simulink library "bcm"  (R2021b)
settings: Solver=VariableStepAuto  StartTime=0.0  StopTime=10.0  RelTol=1e-3
undefined symbols (not defined in the file): ENUM_ANTITHEFT_ALARM, ENUM_ANTITHEFT_ARM, ENUM_ANTITHEFT_DISARM, ENUM_ANTITHEFT_WAIT, ENUM_GEARPOSNTOCAN_P, ENUM_PDKEYRAWLULOCK_INUNLOCK, ENUM_PDKEYRAWPS_INPS, ENUM_POWERSTA_ON, ENUM_POWERSTA_READY, ENUM_POWERSTA_STANDBY, ENUM_PWRSTASW_ON, ENUM_PWRSTASW_READY, ENUM_SYSMODE_DEVELOPING, ENUM_SYSMODE_PRODUCT, ENUM_VEHICLETYPE_D21, ENUM_VEHICLETYPE_D31F25, ENUM_VEHICLETYPE_D31HAWD, ENUM_VEHICLETYPE_D31HRWD, ENUM_VEHICLETYPE_D31L24, FALSE, KBCM_ACCSwcPrsTmr_s, KBCM_ALMBrightnessDark_enum, KBCM_AmbBlue_enum, KBCM_AmbBreathT_ms, KBCM_AmbGreen_enum, KBCM_AmbMidPple_enum, KBCM_AmbRed_enum, KBCM_AmbTempCtrlEN_flg, KBCM_AmbTempT_s, KBCM_AmbWelModeENWait_s, KBCM_Antitheft_enum_ovrdflg, KBCM_Antitheft_enum_ovrdval, KBCM_APMDoorCtrlSta_flg_ovrdflg, KBCM_APMDoorCtrlSta_flg_ovrdval, KBCM_CmdKeepT_s, KBCM_CSWLightRstDebT_s, KBCM_CSWTurnLPRstT_s, KBCM_CycleTimeSet_s, KBCM_DelayTSW_flg, KBCM_DiagDRLOFF_flg, KBCM_DiagFLTC_mA, KBCM_DiagFMHT_s, KBCM_DiagFRTC_mA, KBCM_DiagRLTC_mA, KBCM_DiagRRTC_mA, KBCM_DrAPMRetryTimes_cnt, KBCM_DrOpenWdwOT_s, KBCM_DrOpenWdwReady_s, KBCM_DutyCycleSet_cnt, KBCM_DutyOverride_flg, KBCM_DutyOverride_val, KBCM_ESSOffT_ms, KBCM_ESSOnT_ms, KBCM_FDCDKCReDetectT_K, KBCM_FDCDKCUSSFilterT_K, KBCM_HandleLampKeepT_s, KBCM_IVIRstHoldT_ms, KBCM_IVIRstTriggerT_ms, KBCM_ONDelayT_ms, KBCM_RAPSAbnFlashOFFT_ms ... (+51)
libraries: simulink x402, $bdroot x10, hcu_lib x2
(part 12 of 14)

== stateflow chart bcm/BCM/BCM/AntiTheft/Chart ==
  settings: sampleTime=StepSize
  state AlertTone [parallel]
    settings: executionOrder=11
    state OFF
      en:VBCM_LockAlarm_enum=0;
    state Lock_Success
      en:VBCM_LockAlarm_enum=1;
    (default) -> AlertTone.OFF
    Lock_Success -> AlertTone.OFF : [after(5,tick)]
    AlertTone -> Lock_Success : eLockAlert [IVI_Lock_SoundSW_Sta==1]
  state HoodRelease [parallel]
    settings: executionOrder=12
    state OFF
      en:FDC_BCM_HoodRel_Cmd=0;
    state Hood_Release
      en:FDC_BCM_HoodRel_Cmd=1;
    (default) -> HoodRelease.OFF
    (junction 2202) -> HoodRelease.OFF
    HoodRelease -> Hood_Release [order 1] : eHoodRel
        | [VehSpeed<=0 && ShiftGearPosn == ENUM_GEARPOSNTOCAN_P]
    Hood_Release -> (junction 2202) : [after(10,tick)]
    HoodRelease -> Hood_Release [order 2] : [VBCM_IVIFrTrunkUnlockReqRising_flg && ....
        | (VehSpeed<=0 && ShiftGearPosn == ENUM_GEARPOSNTOCAN_P && !DrLockSta)]
  state ATLockCtrl [parallel]
    settings: executionOrder=6
    state Lock
      en:ATLockCtrl=1;
    state StandBy
      en:ATLockCtrl=0;
    note: 350 ms
    state Unlock
      en:ATLockCtrl=2;
    (default) -> ATLockCtrl.StandBy
    ATLockCtrl.StandBy -> ATLockCtrl.Lock [order 1] : eActLock
    ATLockCtrl.Lock -> ATLockCtrl.StandBy : [after(35,tick)]
    ATLockCtrl.Unlock -> ATLockCtrl.Lock [order 2] : eActLock
    ATLockCtrl.StandBy -> ATLockCtrl.Unlock [order 2] : eActUnlock
    ATLockCtrl.Unlock -> ATLockCtrl.StandBy [order 1] : [after(35,tick)]
  state Main [parallel]
    settings: executionOrder=1
    state sDisarm
      en:AntitheftSta=0;
      fFirst=1;
    state sSecurity
      state sSecurity
        en:
        AntitheftSta=1;
        fFirst=0;
      note: 28 sec
      note: 10 times
      state sAlarm
        en:
        AntitheftSta=3;
        ATAlarm=1;
        Horn.eHornAlarm;
        CountAlarm=CountAlarm+1;
        ex:ATAlarm=0;
      (junction 1705) -> (junction 1971) [order 2] : {Horn.eHornLock;}
      (junction 1705) -> Main.sSecurity.sSecurity [order 1] : [fHornOFF==1||fFirst==1]
          | /{fHornOFF=0;AlertTone.eLockAlert;}
      (junction 1971) -> Main.sSecurity.sSecurity
      Main.sSecurity.sSecurity -> sAlarm : eDoorOpen[CountAlarm<10]
      sAlarm -> Main.sSecurity.sSecurity : [after(2800,tick)]
    note: 1 sec
    state sLockCheck
    (default) -> (junction 2132) : {CountAlarm = VINP_FlashCountAlarm_enum;}
    (junction 2132) -> (junction 2133) [order 1]
    (junction 2133) -> (junction 2135) [order 1]
    (junction 2132) -> sDisarm [order 2]
    (junction 2133) -> Main.sSecurity.sSecurity [order 2] : [VBCM_FlashAntitheft_enum == ENUM_ANTITHEFT_ARM]
    (junction 2135) -> sAlarm : [VBCM_FlashAntitheft_enum == ENUM_ANTITHEFT_ALARM]
    (junction 1713) -> sDisarm : {ATLockCtrl.eActUnlock;Horn.eLockFail;}
    (junction 1703) -> (junction 1713) [order 1] : [!DrLockSta||AllDoorSW||TailgateSW||HoodSW]
    (junction 1703) -> (junction 1705) [order 2] : {CountAlarm=0;}
    (junction 1686) -> (junction 1713) [order 1] : [AllDoorSW||TailgateSW||HoodSW]
    sLockCheck -> (junction 1703) : [after(100,tick)]
    sDisarm -> sDisarm [order 2] : eUnlock{ATCtrl.eLampUnlock;ATLockCtrl.eActUnlock;}
    (junction 1686) -> sLockCheck [order 2] : {ATLockCtrl.eActLock;}
    (junction 1712) -> (junction 1686) : {ATCtrl.eLampLock;}
    sDisarm -> (junction 1712) [order 1] : eLock
    Main.sSecurity -> (junction 1712) [order 2] : eLock
    Main.sSecurity -> sDisarm [order 1] : eUnlock{ATCtrl.eLampUnlock;ATLockCtrl.eActUnlock;}
    Main.sSecurity -> sDisarm [order 3] : eForceDisarm
  state DKCCmd [parallel]
    settings: executionOrder=2
    state WaitForZone
    state Lock
      en:Main.eLock;
    state Unlock
      en:Main.eUnlock;
    state sStandBy
    state Tailgate
      en:DoorSWDetection.TailgateSW.eTailgate;
      PowerTailgate.eTailgateRemote;
    state FindCar
      en:Horn.eHornLock;ATCtrl.eLampUnlock;
    state TailgateLockFail
      en:Horn.eLockFail;Main.eUnlock;
    state TailgateHandle
      en:DoorSWDetection.TailgateSW.eTailgate;
      PowerTailgate.eTailgateHandle;
    state ForceDisarm
      en:Main.eForceDisarm;
    state FindCarMute
      en:ATCtrl.eLampUnlock;
    state HoodRel
      en:HoodRelease.eHoodRel;
      DoorSWDetection.HoodSW.eHoodRemote;
    DKCCmd -> (junction 2148) : [hasChanged(P_CommandtoBCM)]{PcmdBuf=P_CommandtoBCM;}
    (junction 2148) -> DKCCmd.WaitForZone [order 2]
    (junction 2148) -> (junction 2154) [order 1]
    DKCCmd.WaitForZone -> (junction 2154) [order 2]
    (junction 2154) -> (junction 2045) : [VINP_CANMsgValidGWZoneDR1_flg&&VINP_CANMsgValidGWZoneFR1_flg && Loadbar]
    DKCCmd.WaitForZone -> (junction 2151) [order 1] : [after(150,tick)]
    (junction 2151) -> (junction 2045)
    (junction 2045) -> (junction 2170) [order 1] : [VehSpeed<=0]
    (junction 2170) -> DKCCmd.Lock [order 1] : [PcmdBuf==1]
    (junction 2045) -> (junction 2046) [order 2]
    (junction 2170) -> (junction 2172) [order 2]
    (junction 2172) -> DKCCmd.Lock [order 1] : [PcmdBuf==10 &&....
        | FDC_BCM_WalkOutLkEnFun_Sta==1]
    (junction 2172) -> (junction 2178) [order 2]
    (junction 2178) -> (junction 2180) [order 1] : [PcmdBuf==9]
    (junction 2180) -> DKCCmd.Lock [order 1] : [AntitheftSta==0]
    (junction 2178) -> (junction 2186) [order 2]
    (junction 2180) -> (junction 2183) [order 2]
    (junction 2183) -> DKCCmd.Unlock
    (junction 2186) -> DKCCmd.Unlock [order 1] : [PcmdBuf==11 &&....
        | FDC_BCM_WalkInUnLkEnFun_Sta==1]
    (junction 2186) -> (junction 2189) [order 2]
    (junction 2189) -> DKCCmd.Unlock : [PcmdBuf==2]
    (junction 2046) -> DKCCmd.Unlock [order 1] : [VehSpeed<=0&&PcmdBuf==2]
    (junction 2046) -> (junction 2047) [order 2]
    (default) -> DKCCmd.sStandBy : {PcmdBuf=0;}
    (junction 2047) -> DKCCmd.Tailgate [order 1] : [PcmdBuf==3]
    (junction 2047) -> (junction 2048) [order 2]
    (junction 2048) -> DKCCmd.FindCar [order 1] : [PcmdBuf==4]
    (junction 2048) -> (junction 2049) [order 2]
    (junction 2049) -> TailgateLockFail [order 1] : [PcmdBuf==5]
    (junction 2049) -> (junction 2050) [order 2]
    (junction 2050) -> DKCCmd.TailgateHandle [order 1] : [PcmdBuf==6]
    (junction 2050) -> (junction 2108) [order 2]
    (junction 2108) -> ForceDisarm [order 1] : [PcmdBuf==7]
    (junction 2108) -> (junction 2124) [order 2]
    (junction 2124) -> DKCCmd.FindCarMute [order 1] : [PcmdBuf==8]
    (junction 2124) -> (junction 2193) [order 2]
    (junction 2193) -> DKCCmd.sStandBy [order 2]
    (junction 2193) -> DKCCmd.HoodRel [order 1] : [PcmdBuf==12]
  state Horn [parallel]
    settings: executionOrder=3
    state sStandBy
      en:HornCtrl=0;
    note: 250 ms
    state sAlarm2
      en:HornCtrl=0;
    state sAlarm1
      en:HornCtrl=1;
    state sLock
      en:HornCtrl=1;
    state sKeyIN1
      en:HornCtrl=1;
    state sKeyIN2
      en:HornCtrl=0;
    state sLockFail1
      en:HornCtrl=1;
    state sLockFail2
      en:HornCtrl=0;
    state sLockFail3
      en:HornCtrl=1;
    state sRAPSAlarm2
      en:HornCtrl=0;
    state sRAPSAlarm1
      en:HornCtrl=1;
    (default) -> Horn.sStandBy
    (junction 2243) -> Horn.sStandBy
    sAlarm1 -> sAlarm2 : [after(25,tick)]
    sAlarm2 -> (junction 2243) [order 1] : [ATAlarm==0]
    Horn -> sAlarm1 [order 1] : eHornAlarm
    (junction 2244) -> (junction 2243)
    sAlarm2 -> sAlarm1 [order 2] : [after(25,tick)]
    sLock -> (junction 2244) : [after(3,tick)]
    (junction 2245) -> (junction 2244)
    Horn -> sLock [order 2] : eHornLock
    sKeyIN2 -> sLock : [after(5,tick)]
    Horn -> sKeyIN1 [order 3] : eKeyIN
    sKeyIN1 -> sKeyIN2 : [after(3,tick)]
    Horn -> sLockFail1 [order 4] : eLockFail
    sLockFail1 -> sLockFail2 : [after(10,tick)]
    sLockFail2 -> sLockFail3 : [after(30,tick)]
    sLockFail3 -> (junction 2245) : [after(10,tick)]
    (junction 2246) -> (junction 2245)
    sRAPSAlarm1 -> sRAPSAlarm2 : [after(25,tick)]
    sRAPSAlarm2 -> (junction 2246) [order 2] : [RAPSHornReq==0]
    Horn -> sRAPSAlarm1 [order 5] : eRAPSHorn
    sRAPSAlarm2 -> sRAPSAlarm1 [order 1] : [after(25,tick)]
  state DoorSWDetection [parallel]
    settings: executionOrder=4
    state DrDoor [parallel]
      settings: executionOrder=1
      state DrDoorSW_Open
      state DrDoorSW_Close
      (default) -> DrDoorSW_Open
      DrDoorSW_Open -> DrDoorSW_Close : [!DrDoorSW]
      DrDoorSW_Close -> DrDoorSW_Open : [DrDoorSW]/{Main.eDoorOpen;}
    state PsDoor [parallel]
      settings: executionOrder=2
      state PsDoorSW_Open
      state PsDoorSW_Close
      (default) -> PsDoorSW_Open
      PsDoorSW_Open -> PsDoorSW_Close : [!PsDoorSW]
      PsDoorSW_Close -> PsDoorSW_Open : [PsDoorSW]/{Main.eDoorOpen;}
    state RLDoor [parallel]
      settings: executionOrder=3
      state RLDoorSW_Open
      state RLDoorSW_Close
      (default) -> RLDoorSW_Open
      RLDoorSW_Open -> RLDoorSW_Close : [!RLDoorSW]
      RLDoorSW_Close -> RLDoorSW_Open : [RLDoorSW]/{Main.eDoorOpen;}
    state RRDoor [parallel]
      settings: executionOrder=4
      state RRDoorSW_Open
      state RRDoorSW_Close
      (default) -> RRDoorSW_Open
      RRDoorSW_Open -> RRDoorSW_Close : [!RRDoorSW]
      RRDoorSW_Close -> RRDoorSW_Open : [RRDoorSW]/{Main.eDoorOpen;}
    state HoodSW [parallel]
      settings: executionOrder=6
      state HoodSW_Open
      state HoodSW_Close
      state sRemote
      state Wait
      state Ignore
      (default) -> HoodSW_Open
      HoodSW_Open -> HoodSW_Close : [!HoodSW]
      HoodSW_Close -> HoodSW_Open [order 1] : [HoodSW]/{Main.eDoorOpen;}
      HoodSW_Close -> DoorSWDetection.HoodSW.sRemote [order 2] : eHoodRemote
      (junction 2220) -> HoodSW_Close [order 2] : [after(2000,tick)]
      Wait -> HoodSW_Close [order 2] : after(100,tick)
      DoorSWDetection.HoodSW.sRemote -> (junction 2220)
      (junction 2220) -> DoorSWDetection.HoodSW.Ignore [order 1] : [HoodSW]
      Wait -> DoorSWDetection.HoodSW.Ignore [order 1] : [HoodSW]
      DoorSWDetection.HoodSW.Ignore -> Wait : [!HoodSW]
    note: 20 sec
    state TailgateSW [parallel]
      settings: executionOrder=5
      state TailgateSW_Open
      state TailgateSW_Close
      state sRemote
      state Ignore
      (default) -> TailgateSW_Open
      TailgateSW_Open -> TailgateSW_Close : [!TailgateSW]
      TailgateSW_Close -> TailgateSW_Open [order 1] : [TailgateSW]/{Main.eDoorOpen;}
      TailgateSW_Close -> DoorSWDetection.TailgateSW.sRemote [order 2] : eTailgate
      (junction 1886) -> TailgateSW_Close [order 2] : [after(1500,tick)]
      DoorSWDetection.TailgateSW.Ignore -> TailgateSW_Close : [!TailgateSW]
      DoorSWDetection.TailgateSW.sRemote -> (junction 1886)
      (junction 1886) -> DoorSWDetection.TailgateSW.Ignore [order 1] : [TailgateSW]
    note: 15 sec
  state VIGCommand [parallel]
    settings: executionOrder=7
    state WaitForZone
    state StandBy
    state Lock
      en:Main.eLock;
    state Unlock
      en:Main.eUnlock;
    state FindCar
      en:Horn.eHornLock;ATCtrl.eLampUnlock;
    state FindCarMute
      en:ATCtrl.eLampUnlock;
    state Tailgate
      en:DoorSWDetection.TailgateSW.eTailgate;
      PowerTailgate.eTailgateRemote;
    state TailgateReject
      en:PowerTailgate.eTailgateReject;
    state HoodRel
      en:HoodRelease.eHoodRel;
      DoorSWDetection.HoodSW.eHoodRemote;
    (default) -> VIGCommand.WaitForZone
    VIGCommand.WaitForZone -> VIGCommand.StandBy : [VINP_CANMsgValidGWZoneDR1_flg&&VINP_CANMsgValidGWZoneFR1_flg]
    VIGCommand.StandBy -> VIGCommand.Lock [order 1] : [VehSpeed<=0&&(VIG_Cmd==1||VIG_Cmd==5)]
    VIGCommand.Lock -> VIGCommand.StandBy : [VIG_Cmd==0]
    (junction 1941) -> VIGCommand.Lock [order 1] : [AntitheftSta==0||AntitheftSta==2]/{fHornOFF=1;}
    VIGCommand.StandBy -> (junction 1941) [order 6] : [VehSpeed<=0&&VIG_Cmd==7]
    (junction 1941) -> VIGCommand.Unlock [order 2] : [fVIGHandle==0]
    VIGCommand.StandBy -> VIGCommand.Unlock [order 2] : [VehSpeed<=0&&(VIG_Cmd==2||VIG_Cmd==6)]
    VIGCommand.Unlock -> VIGCommand.StandBy : [VIG_Cmd==0]
    VIGCommand.StandBy -> VIGCommand.FindCar [order 3] : [VIG_Cmd==3]
    VIGCommand.FindCar -> VIGCommand.StandBy : [VIG_Cmd==0]
    VIGCommand.StandBy -> VIGCommand.FindCarMute [order 5] : [VIG_Cmd==8]
    VIGCommand.FindCarMute -> VIGCommand.StandBy : [VIG_Cmd==0]
    VIGCommand.Tailgate -> VIGCommand.StandBy : [VIG_Cmd==0]
    (junction 2118) -> VIGCommand.Tailgate
    (junction 2116) -> (junction 2118) [order 2]
    VIGCommand.StandBy -> (junction 2116) [order 4] : [VIG_Cmd==4]
    (junction 2116) -> TailgateReject [order 1] : [PwrSta==5]
    TailgateReject -> VIGCommand.StandBy : [VIG_Cmd==0]
    VIGCommand.StandBy -> VIGCommand.HoodRel [order 7] : [VIG_Cmd==11]
    VIGCommand.HoodRel -> VIGCommand.StandBy : [VIG_Cmd==0]
  state PowerTailgate [parallel]
    settings: executionOrder=9
    state StandBy
      en:TailgateRemote=0;
    state TailgateRemote
      en:TailgateRemote=1;
    note: 200 ms
    state TailgateHandle
      en:TailgateRemote=2;
    note: 200 ms
    state TailgateHandle1
      en:TailgateRemote=3;
    (default) -> PowerTailgate.StandBy
    PowerTailgate.StandBy -> TailgateRemote [order 1] : eTailgateRemote
    TailgateRemote -> PowerTailgate.StandBy : [after(20,tick)]
    PowerTailgate.StandBy -> PowerTailgate.TailgateHandle [order 2] : eTailgateHandle
    PowerTailgate.TailgateHandle -> PowerTailgate.StandBy : [after(20,tick)]
    PowerTailgate.StandBy -> TailgateHandle1 [order 3] : eTailgateReject
    TailgateHandle1 -> PowerTailgate.StandBy : [after(20,tick)]
  state AGSTailgateOpen [parallel]
    settings: executionOrder=8
    state sStandBy
    state Tailgate
      en:DoorSWDetection.TailgateSW.eTailgate;
      PowerTailgate.eTailgateRemote;
    (default) -> AGSTailgateOpen.sStandBy
    AGSTailgateOpen.sStandBy -> AGSTailgateOpen.Tailgate : [APSOpenPTG==1&&TailgateSW==0]
    AGSTailgateOpen.Tailgate -> AGSTailgateOpen.sStandBy : [APSOpenPTG==0]
  state AntitheftSeat [parallel]
    settings: executionOrder=10
    state StandBy
      en:AntitheftSeatFlod=0;
    state Lock_Check
      en:AntitheftSeatFlod=0;
    state Flod
      en:AntitheftSeatFlod=1;
    note: 200 ms
    (default) -> AntitheftSeat.StandBy
    AntitheftSeat.StandBy -> Lock_Check : [fHornOFF==1]
    Lock_Check -> Flod : [fHornOFF==0]
    Flod -> Lock_Check [order 2] : [fHornOFF==1]
    Flod -> AntitheftSeat.StandBy [order 1] : [after(20,tick)]
  state RAPS_Lock_Request [parallel]
    settings: executionOrder=13
    state NOReq
    state LOCK
      en:Main.eLock;
    (default) -> RAPS_Lock_Request.NOReq
    RAPS_Lock_Request.NOReq -> LOCK : [hasChanged(RAPSBCMLockReqCmd) &&....
        | RAPSBCMLockReqCmd &&....
        | PwrSta>3]
    LOCK -> RAPS_Lock_Request.NOReq : [!RAPSBCMLockReqCmd]
  state RAPS_Horn [parallel]
    settings: executionOrder=14
    state NoRequest
      en:
      RAPSHornReq=0;
    state RAPS_HornReq
      en:
      Horn.eRAPSHorn;
      RAPSHornReq=1;
    (default) -> NoRequest
    NoRequest -> RAPS_HornReq : [DrSeatSta!=1 && hasChanged(RAPSErrWarn) && RAPSErrWarn==2]
    RAPS_HornReq -> NoRequest : [DrSeatSta==1 || RAPSErrWarn!=2 || after(2800,tick)]
  state RAPS_UnLock_Request [parallel]
    settings: executionOrder=15
    state NOReq
    state UNLOCK
      en:Main.eUnlock;
    (default) -> RAPS_UnLock_Request.NOReq
    RAPS_UnLock_Request.NOReq -> UNLOCK : [RAPS_Unlock_Req]
    UNLOCK -> RAPS_UnLock_Request.NOReq : [!RAPS_Unlock_Req]
  state ATCtrl [parallel]
    settings: executionOrder=5
    state StandBy
      en:ATCtrl=0;
    state Lock
      en:ATCtrl=1;
    note: 350 ms
    state Unlock
      en:ATCtrl=2;
    (default) -> ATCtrl.StandBy
    ATCtrl.StandBy -> ATCtrl.Lock [order 1] : eLampLock
    ATCtrl.Lock -> ATCtrl.StandBy [order 1] : [after(35,tick)]
    ATCtrl.Unlock -> ATCtrl.Lock [order 2] : eLampLock
    ATCtrl.Lock -> ATCtrl.Unlock [order 2] : eLampUnlock
    ATCtrl.StandBy -> ATCtrl.Unlock [order 2] : eLampUnlock
    ATCtrl.Unlock -> ATCtrl.StandBy [order 1] : [after(35,tick)]
  data: P_CommandtoBCM input uint8 [0..11]; PwrSta input uint8 [0..5]; ATCtrl output uint8; ATLockCtrl output uint8; AllDoorSW input boolean [0..1]; HoodSW input boolean; TailgateSW input boolean; DrDoorSW input boolean; PsDoorSW input boolean; RLDoorSW input boolean; RRDoorSW input boolean; DrLockSta input boolean; ATAlarm output boolean; AntitheftSta output uint8; TailgateRemote output uint8; HornCtrl output boolean; VIG_Cmd input uint8 [0..7]; VehSpeed input single [0..1]; fVIGHandle input boolean; VBCM_FlashAntitheft_enum input uint8; fFirst local boolean; fHornOFF local boolean; AntitheftSeatFlod output boolean; APSOpenPTG input boolean; ENUM_ANTITHEFT_ALARM parameter uint8; ENUM_ANTITHEFT_ARM parameter uint8; VINP_FlashCountAlarm_enum input uint8; VINP_CANMsgValidGWZoneDR1_flg input boolean; VINP_CANMsgValidGWZoneFR1_flg input boolean; PcmdBuf local uint8; CountAlarm output uint8; IVI_Lock_SoundSW_Sta input boolean; FDC_BCM_WalkOutLkEnFun_Sta input; FDC_BCM_WalkInUnLkEnFun_Sta input; VBCM_LockAlarm_enum output uint8; Loadbar input; ShiftGearPosn input; FDC_BCM_HoodRel_Cmd output boolean; VBCM_IVIFrTrunkUnlockReqRising_flg input; ENUM_GEARPOSNTOCAN_P parameter; DrSeatSta input; RAPSBCMLockReqCmd input; RAPSErrWarn input; RAPSHornReq local boolean; RAPS_Unlock_Req input
  data PwrSta settings: description=Min=0, Max=2047, Engineering Unit = km/h, Offset=0 km/h, Resolution= 0.125 km/h per bit, >2047 = Invalid (bit 12 = 1)
  events: eLockAlert local FUNCTION_CALL_EVENT; eHoodRel local FUNCTION_CALL_EVENT; eActLock local FUNCTION_CALL_EVENT; eActUnlock local FUNCTION_CALL_EVENT; eLock local FUNCTION_CALL_EVENT; eUnlock local FUNCTION_CALL_EVENT; eDoorOpen local FUNCTION_CALL_EVENT; eForceDisarm local FUNCTION_CALL_EVENT; eHornAlarm local FUNCTION_CALL_EVENT; eHornLock local FUNCTION_CALL_EVENT; eKeyIN local FUNCTION_CALL_EVENT; eLockFail local FUNCTION_CALL_EVENT; eRAPSHorn local FUNCTION_CALL_EVENT; eHoodRemote local FUNCTION_CALL_EVENT; eTailgate local FUNCTION_CALL_EVENT; eTailgateRemote local FUNCTION_CALL_EVENT; eTailgateHandle local FUNCTION_CALL_EVENT; eTailgateReject local FUNCTION_CALL_EVENT; eLampLock local FUNCTION_CALL_EVENT; eLampUnlock local FUNCTION_CALL_EVENT

== stateflow chart bcm/BCM/BCM/CenterDoorLock/Chart ==
  settings: updateMethod=DISCRETE
  state CrashDetect [parallel]
    settings: executionOrder=7
    state OFF [commented out]
    state KeyON [commented out]
      state Initial [commented out]
        en:
        CrashDetd=0;
      state sCrash [commented out]
        en:CrashDetd=1;Unlockreq=1;
      note: 750 ms
      state Detect [commented out]
      Initial -> Detect [commented out] : [after(75,tick)]
      Detect -> sCrash [commented out] : [CrashOutputSts>0||....
          | (CrashInputFreq>4.1&&....
          | CrashInputFreq<4.2&&....
          | CrashInputDuty>16&&....
          | CrashInputDuty<17)]
    (default) -> CrashDetect.OFF [commented out]
    CrashDetect.OFF -> Initial [commented out] : [PwrSta>3]
    KeyON -> CrashDetect.OFF [commented out] : [PwrSta<=3]
    (default) -> (junction 1980)
    (junction 1980) -> (junction 1981) : [hasChanged(CrashDetd) && CrashDetd == TRUE]
    CrashDetect -> (junction 1980)
    (junction 1981) -> (junction 1979) : {Unlockreq=1;}
  state ChargingDoor [parallel]
    settings: executionOrder=1
    state ChargingDoorUnlock
      en:FrChargingDoorCtrl=0;
      RrChargingDoorCtrl=0;
      FuelDoorPos=0;
    state U2L
      en:FrChargingDoorCtrl=2;
      RrChargingDoorCtrl=2;
    note: 100ms
    note: 100ms
    state L2U
      en:FrChargingDoorCtrl=1;
      RrChargingDoorCtrl=1;
    state ChargingDoorLock
      en:FrChargingDoorCtrl=0;
      RrChargingDoorCtrl=0;
      FuelDoorPos=1;
    (default) -> (junction 1986)
    (junction 1986) -> (junction 1988) [order 2]
    (junction 1986) -> ChargingDoorUnlock [order 1] : [!EEP_FuelDoorPos]
    (junction 1988) -> ChargingDoorLock
    ChargingDoorUnlock -> U2L : [AntitheftSta==1||AntitheftSta==3]
    L2U -> ChargingDoorUnlock : [after(10,tick)]
    U2L -> ChargingDoorLock : [after(10,tick)]
    ChargingDoorLock -> L2U : [AntitheftSta==0||AntitheftSta==2]
  state IVICentralDoorLockSW [parallel]
    settings: executionOrder=3
    state Release
    state Press
    (default) -> IVICentralDoorLockSW.Press
    IVICentralDoorLockSW.Press -> IVICentralDoorLockSW.Release : [CDL_Unlock_Butt==0&&CDL_Lock_Butt==0]
    IVICentralDoorLockSW.Release -> (junction 1950) [order 1] : [CDL_Lock_Butt==1]
    (junction 1950) -> IVICentralDoorLockSW.Press [order 1] : [BCM_DoorLock_Sta]/{Main.eDUnlock;}
    (junction 1950) -> (junction 1951) [order 2]
    (junction 1951) -> IVICentralDoorLockSW.Press [order 1] : [AllDoorSW]/{Main.eDUnlock;}
    (junction 1951) -> (junction 1952) [order 2]
    (junction 1952) -> IVICentralDoorLockSW.Press [order 1] : [CrashDetd==1]{Main.eDUnlock;}
    (junction 1952) -> (junction 1953) [order 2]
    (junction 1953) -> IVICentralDoorLockSW.Press : {Main.eCTDLock;}
    IVICentralDoorLockSW.Release -> IVICentralDoorLockSW.Press [order 2] : [CDL_Unlock_Butt==1]{Main.eDUnlock;}
  state ATLockCtrl [parallel]
    settings: executionOrder=4
    state LockSend
      en:
      fUnlockSingle=1;
    state NoCommand
    state UnlockSend
      en:fUnlockSingle=0;
    (default) -> NoCommand : {fUnlockSingle=VINP_FlashfUnlockSingle_flg;}
    NoCommand -> (junction 2142) [order 2] : [ATLockCtrl==1....
        | ||....
        | VBCM_AutoLockReq_flg]
    (junction 2142) -> LockSend [order 1] : [CrashDetd==1]
    (junction 2142) -> (junction 2132) [order 2] : {Main.eDLock;}
    (junction 2132) -> LockSend
    LockSend -> NoCommand : [ATLockCtrl!=1]
    NoCommand -> (junction 2143) [order 1] : [ATLockCtrl==2....
        | ||....
        | VBCM_AutoUnlockReq_flg]
    (junction 2143) -> UnlockSend [order 1] : [LockSetting==0||fUnlockSingle==0]/{Main.eDUnlock;}
    (junction 2143) -> (junction 2144) [order 2]
    (junction 2144) -> UnlockSend : /{Main.eSUnlock;}
    UnlockSend -> NoCommand : [ATLockCtrl!=2 && !VBCM_AutoUnlockReq_flg]
  state CentralDoorLockSW [parallel]
    settings: executionOrder=2
    state Release
    state Press
    (default) -> CentralDoorLockSW.Press
    CentralDoorLockSW.Press -> CentralDoorLockSW.Release : [!CentralDoorLockSW]
    CentralDoorLockSW.Release -> (junction 1817) : [CentralDoorLockSW]
    (junction 1817) -> CentralDoorLockSW.Press [order 1] : [BCM_DoorLock_Sta]/{Main.eDUnlock;}
    (junction 1817) -> (junction 1821) [order 2]
    (junction 1821) -> CentralDoorLockSW.Press [order 1] : [AllDoorSW]/{Main.eDUnlock;}
    (junction 1821) -> (junction 1824) [order 2]
    (junction 1824) -> CentralDoorLockSW.Press [order 1] : [CrashDetd==1]{Main.eDUnlock;}
    (junction 1824) -> (junction 1827) [order 2]
    (junction 1827) -> CentralDoorLockSW.Press : {Main.eCTDLock;}
  state AutoFoldforHandle [parallel]
    settings: executionOrder=10
    state sStop
    state sMoving
    (default) -> sStop
    sMoving -> sStop : [VehSpeed <= 0]
    sStop -> (junction 2026) : [VehSpeed >= 10 && VehSpeed < 256]
    (junction 2026) -> sMoving [order 1] : [!CrashDetd && ...
        | (!VINP_FLHandleClose_flg || !VINP_FRHandleClose_flg || ....
        |  !VINP_RLHandleClose_flg || !VINP_RRHandleClose_flg)]
        | {VBCM_FDHandleCmd_enum = 3;
        |  LHandleLampCtrl = 1;
        |  RHandleLampCtrl = 1;}
    (junction 2026) -> (junction 2027) [order 2]
    (junction 2027) -> sMoving
  state LED [parallel]
    settings: executionOrder=6
    state OFF
      en:DoorLockIND=0;
    state ON
      en:DoorLockIND=1;
    note: 10 sec
    state HoldON
      en:DoorLockIND=1;
    (default) -> LED.OFF
    ON -> LED.OFF [order 1] : [BCM_DoorLock_Sta==0]
    LED.OFF -> ON [order 1] : [PwrSta>3&&BCM_DoorLock_Sta==1]
    HoldON -> LED.OFF [order 1] : [after(1000,tick)||BCM_DoorLock_Sta==0]
    LED.OFF -> HoldON [order 2] : eResetLED[BCM_DoorLock_Sta==1]
    HoldON -> ON [order 2] : [PwrSta>3]
    ON -> HoldON [order 2] : [PwrSta<=3]
    HoldON -> HoldON [order 3] : eResetLED
  state Main [parallel]
    settings: executionOrder=5
    note: 350 ms
    state WaitForReverse
      en:CTDCtrl=0;
    state StandBy
      en:CTDCtrl=0;
    state DoorLock
      en:CTDCtrl=3;
    note: 100 ms
    state DrDoorUnlock
      en:CTDCtrl=1;
      fVIGHandle=0;
    note: Unlockreq
    state DoorUnlock
      en:CTDCtrl=2;
      fVIGHandle=0;
      ex:Unlockreq=0;
    (default) -> Main.StandBy
    Main.StandBy -> DoorLock [order 1] : eDLock
    DoorLock -> WaitForReverse [order 1] : [after(35,tick)]/{LED.eResetLED;}
    DoorLock -> WaitForReverse [order 2] : [Unlockreq]/{LED.eResetLED;}
    Main.StandBy -> DoorLock [order 5] : eCTDLock{fVIGHandle=1;}
    WaitForReverse -> Main.StandBy : [after(10,tick)]
    Main.StandBy -> DrDoorUnlock [order 2] : eSUnlock
    DrDoorUnlock -> WaitForReverse [order 1] : [after(35,tick)]
    DrDoorUnlock -> DoorUnlock [order 2] : eDUnlock
    DrDoorUnlock -> DoorUnlock [order 3] : [Unlockreq]
    DoorUnlock -> WaitForReverse : [after(35,tick)]
    Main.StandBy -> DoorUnlock [order 3] : eDUnlock
    Main.StandBy -> DoorUnlock [order 4] : [Unlockreq]
  state LHandleLampPowerCtrlforHandle [parallel]
    settings: executionOrder=12
    state sKeep
      en:
      VBCM_FDLHandleLampCmd_flg = 1;
    state sStandBy
      en:
      VBCM_FDLHandleLampCmd_flg = 0;
      LHandleLampCtrl = 0;
    LHandleLampPowerCtrlforHandle -> LHandleLampPowerCtrlforHandle.sKeep : [hasChanged(VBCM_FDHandleCmd_enum) && ...
        | (VBCM_FDHandleCmd_enum == 1 || ...
        |  VBCM_FDHandleCmd_enum == 2)]
    LHandleLampPowerCtrlforHandle.sKeep -> LHandleLampPowerCtrlforHandle.sStandBy : [after (KBCM_HandleLampKeepT_s, tick) || ...
        | (LHandleLampCtrl && ...
        |  VINP_FLHandleClose_flg)]
    (default) -> LHandleLampPowerCtrlforHandle.sStandBy
  state DoorOpenDetectforHandle [parallel]
    settings: executionOrder=8
    state sDrDoorOpenDet [parallel]
      settings: executionOrder=1
      (default) -> (junction 2039)
      sDrDoorOpenDet -> (junction 2038) : [hasChanged(VINP_DrDoorSW_flg) && VINP_DrDoorSW_flg]
      (junction 2038) -> (junction 2039) : [VehSpeed <= 0 && VINP_FLHandleClose_flg]
          | {VBCM_FDHandleCmd_enum = 1;
          |  LHandleLampCtrl = 0;}
    state sPsDoorOpenDet [parallel]
      settings: executionOrder=2
      (default) -> (junction 2045)
      (junction 2044) -> (junction 2045) : [VehSpeed <= 0 && ...
          | (VINP_FLHandleClose_flg || VINP_FRHandleClose_flg)]
          | {VBCM_FDHandleCmd_enum = 2;
          |  RHandleLampCtrl = 0;}
      sPsDoorOpenDet -> (junction 2044) : [hasChanged(VINP_PsDoorSW_flg) && VINP_PsDoorSW_flg]
    state sRLDoorOpenDet [parallel]
      settings: executionOrder=3
      (default) -> (junction 2051)
      sRLDoorOpenDet -> (junction 2050) : [hasChanged(VINP_RLDoorSW_flg) && VINP_RLDoorSW_flg]
      (junction 2050) -> (junction 2051) : [VehSpeed <= 0 && ...
          | (VINP_FLHandleClose_flg || VINP_RLHandleClose_flg)]
          | {VBCM_FDHandleCmd_enum = 2;
          |  RHandleLampCtrl = 0;}
    state sRRDoorOpenDet [parallel]
      settings: executionOrder=4
      (default) -> (junction 2057)
      sRRDoorOpenDet -> (junction 2056) : [hasChanged(VINP_RRDoorSW_flg) && VINP_RRDoorSW_flg]
      (junction 2056) -> (junction 2057) : [VehSpeed <= 0 && ...
          | (VINP_FLHandleClose_flg || VINP_RRHandleClose_flg)]
          | {VBCM_FDHandleCmd_enum = 2;
          |  RHandleLampCtrl = 0;}
  state AutoLock [parallel]
    settings: executionOrder=14
    state StandBy
      en:
      VBCM_AutoUnlockReq_flg = 0;
      VBCM_AutoLockReq_flg = 0;
    state AutoLock
      en:
      VBCM_AutoLockReq_flg = 1;
      VBCM_AutoLockDisable_flg = 1;
    state AutoUnlock
      en:
      VBCM_AutoUnlockReq_flg = 1;
      VBCM_AutoLockDisable_flg = 0;
    state AutoLockENRst
      en:
      VBCM_AutoLockDisable_flg = 0;
    (default) -> AutoLock.StandBy
    AutoLock.StandBy -> AutoLock.AutoLock [order 3] : [AirBagFailCmd==0 && CrashDetd==0 && VehSpeed>=10 && VehSpeed<=240 && VBCM_AutoLockSta_flg && !VBCM_AutoLockDisable_flg]
    AutoLock.AutoLock -> AutoLock.StandBy
    AutoLock.StandBy -> AutoUnlock [order 1] : [VBCM_AutoUnlockSta_flg && ShiftGearPosnBuf != 0 && VTQD_ShiftGearPosn_enum == 0]
    AutoUnlock -> AutoLock.StandBy
    AutoLock.StandBy -> AutoLockENRst [order 2] : [(hasChanged(AllDoorSW) && AllDoorSW == 1)....
        | ||....
        | (PwrStaBuf == 4 || PwrStaBuf == 5) && (PwrSta >= 0 && PwrSta <= 3)....
        | ||....
        | (hasChanged(VBCM_AutoLockSta_flg) && VBCM_AutoLockSta_flg)]
    AutoLockENRst -> AutoLock.StandBy
  state RHandleLampPowerCtrlforHandle [parallel]
    settings: executionOrder=13
    state sKeep
      en:
      VBCM_FDRHandleLampCmd_flg = 1;
    state sStandBy
      en:
      VBCM_FDRHandleLampCmd_flg = 0;
      RHandleLampCtrl = 0;
    RHandleLampPowerCtrlforHandle -> RHandleLampPowerCtrlforHandle.sKeep : [hasChanged(VBCM_FDHandleCmd_enum) && ....
        | VBCM_FDHandleCmd_enum == 2]
    RHandleLampPowerCtrlforHandle.sKeep -> RHandleLampPowerCtrlforHandle.sStandBy : [after (KBCM_HandleLampKeepT_s, tick) || ...
        | (RHandleLampCtrl && ...
        |  VINP_FRHandleClose_flg &&....
        |  VINP_RLHandleClose_flg &&....
        |  VINP_RRHandleClose_flg)]
    (default) -> RHandleLampPowerCtrlforHandle.sStandBy
  state CmdReset [parallel]
    settings: executionOrder=11
    state sKeep
    state sStandBy
      en:
      VBCM_FDHandleCmd_enum = 0;
    CmdReset -> CmdReset.sKeep : [hasChanged(VBCM_FDHandleCmd_enum) && ...
        | VBCM_FDHandleCmd_enum > 0]
    CmdReset.sKeep -> CmdReset.sStandBy : [after (KBCM_CmdKeepT_s, tick)]
    (default) -> CmdReset.sStandBy
  state CTDDoorCtrlforHandle [parallel]
    settings: executionOrder=9
    (default) -> (junction 2009)
    (junction 2008) -> (junction 2009) [order 1] : [VehSpeed <= 0 && CTDCtrl == 1]
        | {VBCM_FDHandleCmd_enum = CTDCtrl;
        |  LHandleLampCtrl = 0;}
    CTDDoorCtrlforHandle -> (junction 2008) : [hasChanged(CTDCtrl) && CTDCtrl > 0]
    (junction 2008) -> (junction 2010) [order 2]
    (junction 2010) -> (junction 2011) [order 1] : [VehSpeed <= 0 && CTDCtrl == 2]
        | {VBCM_FDHandleCmd_enum = CTDCtrl;
        |  LHandleLampCtrl = 0;
        |  RHandleLampCtrl = 0;}
    (junction 2010) -> (junction 2012) [order 2] : [VehSpeed <= 0 && CTDCtrl == 3]
        | {VBCM_FDHandleCmd_enum = CTDCtrl;
        |  LHandleLampCtrl = 1;
        |  RHandleLampCtrl = 1;}
  data: AntitheftSta input uint8 [..3]; FrChargingDoorCtrl output uint8 [0..2]; RrChargingDoorCtrl output uint8 [0..2]; AllDoorSW input boolean; PwrSta input uint8 [0..5]; CentralDoorLockSW input boolean; BCM_DoorLock_Sta input boolean; CTDCtrl output uint8 [0..3]; DoorLockIND output boolean; ATLockCtrl input uint8 [0..2]; AirBagFailCmd input boolean; VehSpeed input; fVIGHandle output boolean; CDL_Unlock_Butt input boolean; CDL_Lock_Butt input boolean; Unlockreq local boolean; CrashDetd input boolean; FuelDoorPos output; EEP_FuelDoorPos input; fUnlockSingle output boolean; VINP_FlashfUnlockSingle_flg input; KBCM_CmdKeepT_s input; KBCM_HandleLampKeepT_s input; VINP_DrDoorSW_flg input; VINP_FLHandleClose_flg input; VINP_FRHandleClose_flg input; VINP_PsDoorSW_flg input; VINP_RLDoorSW_flg input; VINP_RLHandleClose_flg input; VINP_RRDoorSW_flg input; VINP_RRHandleClose_flg input; VBCM_FDLHandleLampCmd_flg output boolean; VBCM_FDRHandleLampCmd_flg output boolean; LHandleLampCtrl local boolean; RHandleLampCtrl local boolean; VBCM_FDHandleCmd_enum output uint8; LockSetting input =0; PwrStaBuf input; ShiftGearPosnBuf input; VBCM_AutoLockSta_flg input; VBCM_AutoUnlockSta_flg input; VTQD_ShiftGearPosn_enum input; VBCM_AutoLockDisable_flg local boolean; VBCM_AutoUnlockReq_flg local boolean; TRUE parameter; VBCM_AutoLockReq_flg local boolean
  events: eResetLED local FUNCTION_CALL_EVENT; eDLock local FUNCTION_CALL_EVENT; eDUnlock local FUNCTION_CALL_EVENT; eSUnlock local FUNCTION_CALL_EVENT; eCTDLock local FUNCTION_CALL_EVENT

== stateflow chart bcm/BCM/BCM/Dimmer/Chart ==
  settings: sampleTime=StepSize
  state CANDimmerCMD [parallel]
    settings: executionOrder=1
    state sWait
    (default) -> sWait
    (junction 1680) -> sWait : [MFRD_N_Bright_Req<=100&&IVI_Status]/{Dimmer=20+MFRD_N_Bright_Req*0.8}
    (junction 1677) -> (junction 1680) [order 1]
    (junction 1677) -> sWait [order 2]
    (junction 1609) -> (junction 1677)
    sWait -> (junction 1609) : [after(20,tick)]
  state sDimmer_EN [parallel]
    settings: executionOrder=2  description=This state models the modes of a door sensor and implements logic to respond when that sensor is producing a signal.
    state sOFF
      en:DimmerEN=0;
    state sON
      en:DimmerEN=1;
    (default) -> sOFF
      settings: description=On the first sample call the door mode is set to active.
    sON -> sOFF : [!PLamp||IVI_Night_Mode_Sta]
    sOFF -> sON : [PLamp&&!IVI_Night_Mode_Sta]
  data: IVI_Status input boolean; IVI_Night_Mode_Sta input boolean; Dimmer output single =0; DimmerEN output boolean; PLamp input boolean; MFRD_N_Bright_Req input =0
  data IVI_Night_Mode_Sta settings: description=Min=0, Max=2047, Engineering Unit = km/h, Offset=0 km/h, Resolution= 0.125 km/h per bit, >2047 = Invalid (bit 12 = 1)
  data Dimmer settings: description=|
      | Bcm Buzzer output results.
      | 0 = None Buzzer
      | 1 = Turn signal Buzzer
      | 2 = Key Reminder Buzzer
      | 3 = Seat Belt Buzzer
      | 4 = Light Monitor Buzzer

== stateflow chart bcm/BCM/BCM/ExteriorLight/Chart ==
  settings: updateMethod=DISCRETE
  state FollowMeSW [parallel]
    settings: executionOrder=2
    state Disabled
    state Enabled
    (default) -> Disabled
    Disabled -> Enabled : [FDC_BCM_FollowMeENFun_Sta==1]
    Enabled -> (junction 2763) [order 2] : [(VBCM_PwrStaBuf_enum==4 || VBCM_PwrStaBuf_enum==5) &&....
        | (VPMM_PwrSta_enum==1 || VPMM_PwrSta_enum==2)]
        | {AutoCut.eFollow;}
    (junction 2763) -> (junction 2765)
    (junction 2755) -> Disabled [order 1] : [VBCM_FollowMe_flg==1]
        | {AutoCut.eFollow;}
    Enabled -> (junction 2755) [order 1] : [FDC_BCM_FollowMeENFun_Sta==0]
    (junction 2755) -> (junction 2758) [order 2]
    (junction 2765) -> Enabled
    (junction 2758) -> Disabled
  state RFogLamp [parallel]
    settings: executionOrder=1
    state sON
      en:VBCM_RrFogLamp_flg=1;
    state sOFF
      en:VBCM_RrFogLamp_flg=0;
    (default) -> RFogLamp.sOFF
    RFogLamp.sOFF -> RFogLamp.sON : [VPMM_PwrSta_enum>3&&....
        | VINP_RFogLampSW_flg==1&&....
        | VBCM_LBeam_flg==1]
    RFogLamp.sON -> RFogLamp.sOFF : [VPMM_PwrSta_enum<=3||....
        | VINP_RFogLampSW_flg==0||....
        | VBCM_LBeam_flg==0]
  state DRL [parallel]
    settings: executionOrder=3
    state sOFF
      en:VBCM_LDRL_flg=0;
      VBCM_RDRL_flg=0;
    state DRL_Opearting
      state sDebounce
      state sON
        en:VBCM_LDRL_flg=1;
        VBCM_RDRL_flg=1;
      note: 300 ms
      state TurnLeft
        en:VBCM_LDRL_flg=0;
        VBCM_RDRL_flg=1;
      state TurnRight
        en:VBCM_LDRL_flg=1;
        VBCM_RDRL_flg=0;
      sDebounce -> (junction 2687) : [after(30,tick)]
      (junction 2687) -> DRL.DRL_Opearting.sON [order 1] : [VBCM_OutMode_enum==0]
      (junction 2687) -> (junction 2689) [order 2]
      DRL.DRL_Opearting.sON -> TurnLeft [order 1] : [VBCM_OutMode_enum==1]
      TurnLeft -> DRL.DRL_Opearting.sON [order 1] : [VBCM_OutMode_enum==0]
      TurnRight -> DRL.DRL_Opearting.sON [order 2] : [VBCM_OutMode_enum==0]
      DRL.DRL_Opearting.sON -> TurnRight [order 2] : [VBCM_OutMode_enum==2]
      (junction 2689) -> TurnLeft [order 1] : [VBCM_OutMode_enum==1]
      (junction 2689) -> (junction 2701) [order 2]
      TurnRight -> TurnLeft [order 1] : [VBCM_OutMode_enum==1]
      TurnLeft -> TurnRight [order 2] : [VBCM_OutMode_enum==2]
      (junction 2701) -> TurnRight
    (default) -> DRL.sOFF
    DRL.sOFF -> sDebounce : [VBCM_DiagDRLOFF_flg==0 &&...
        | VPMM_PwrSta_enum==ENUM_POWERSTA_READY &&...
        | (VTQD_ShiftGearPosn_enum != ENUM_GEARPOSNTOCAN_P || VINP_HeadLampSW_enum==0) &&...
        | !VBCM_PosLamp_flg &&...
        | VBCM_OutMode_enum < 3]
    DRL_Opearting -> DRL.sOFF : [VBCM_DiagDRLOFF_flg==1 ||...
        | VPMM_PwrSta_enum!=ENUM_POWERSTA_READY ||...
        | (VTQD_ShiftGearPosn_enum == ENUM_GEARPOSNTOCAN_P && VINP_HeadLampSW_enum!=0) ||...
        | VBCM_PosLamp_flg ||...
        | VBCM_OutMode_enum >= 3]
  state sBrakeLamp [parallel]
    settings: executionOrder=4
    state sON
      en:VBCM_BrakeLamp_flg=1;
    state sOFF
      en:VBCM_BrakeLamp_flg=0;
    (default) -> sBrakeLamp.sOFF
    sBrakeLamp.sOFF -> sBrakeLamp.sON : [VINP_BrakeSWGPIO_flg==1 || VTQD_ReBrakeLPReq_flg==1 || VINP_ActBrkLampSta_flg==1]
    sBrakeLamp.sON -> sBrakeLamp.sOFF : [VINP_BrakeSWGPIO_flg==0 && VTQD_ReBrakeLPReq_flg==0 && VINP_ActBrkLampSta_flg==0]
  state sReverseLamp [parallel]
    settings: executionOrder=5
    state sON
      en:VBCM_ReverseLamp_flg=1;
    state sOFF
      en:VBCM_ReverseLamp_flg=0;
    (default) -> sReverseLamp.sOFF
    sReverseLamp.sOFF -> sReverseLamp.sON : [VPMM_PwrSta_enum>3&&VTQD_ShiftGearPosn_enum==7]
    sReverseLamp.sON -> sReverseLamp.sOFF : [VPMM_PwrSta_enum<=3||VTQD_ShiftGearPosn_enum!=7]
  state sATCtrl [parallel]
    settings: executionOrder=6
    state StandBy
    state Lock
      en:send(AutoCut.eLock);
    state Unlock
      en:send(AutoCut.eUnlock);
    (default) -> StandBy
    StandBy -> Lock [order 1] : [VBCM_ATCtrl_enum==1]
    Lock -> StandBy : [VBCM_ATCtrl_enum!=1]
    StandBy -> sATCtrl.Unlock [order 2] : [VBCM_ATCtrl_enum==2]
    sATCtrl.Unlock -> StandBy : [VBCM_ATCtrl_enum!=2]
  state PositionLamp [parallel]
    settings: executionOrder=11
    state sPositionLamp
      en:VBCM_PosLamp_flg=1;
    state sOFF
      en:VBCM_PosLamp_flg=0;
    (default) -> PositionLamp.sOFF
    (junction 2636) -> sPositionLamp [order 1] : [VINP_HeadLampSW_enum==1||VINP_HeadLampSW_enum==2]
    PositionLamp.sOFF -> (junction 2636) [order 1] : [!VBCM_AutoCut_flg]
    (junction 2636) -> (junction 2637) [order 2]
    (junction 2637) -> sPositionLamp [order 1] : [VPMM_PwrSta_enum > 3 &&....
        | VINP_HeadLampSW_enum == 0 &&....
        | VINP_RLSLampSta_flg]
    (junction 2637) -> (junction 2638) [order 2]
    (junction 2638) -> sPositionLamp : [VBCM_FollowMe_flg]
    PositionLamp.sOFF -> sPositionLamp [order 2] : [VBCM_showupEN_flg && VBCM_showup_flg]
    (junction 2639) -> PositionLamp.sOFF : [!VBCM_FollowMe_flg &&....
        | (VINP_HeadLampSW_enum == 3 ||....
        | (VINP_HeadLampSW_enum == 0 &&....
        | (VPMM_PwrSta_enum <= 3 || !VINP_RLSLampSta_flg)))]
    (junction 2640) -> (junction 2639) [order 2]
    (junction 2640) -> PositionLamp.sOFF [order 1] : [VBCM_AutoCut_flg]
    sPositionLamp -> (junction 2640) : [!VBCM_showupEN_flg || !VBCM_showup_flg]
  state AutoCut [parallel]
    settings: executionOrder=12
    state FollowMeHome
      en:
      VBCM_FollowMe_flg=1;
      VBCM_AutoCut_flg=0;
      VBCM_showup_flg=0;
      ex:
      VBCM_FollowMe_flg=0;
    state Normal
      state sNormal
        en:VBCM_AutoCut_flg=0;
        VBCM_showup_flg=0;
      state AutoCutDetect
      note: 40 sec
      state Unlock
        en:VBCM_AutoCut_flg=1;
        VBCM_showup_flg=1;
        note: 30 sec
      state AutoCut
        en:VBCM_AutoCut_flg=1;
        VBCM_showup_flg=0;
        VBCM_FollowMe_flg=0;
      sNormal -> AutoCutDetect : [VPMM_PwrSta_enum<=3&&(VINP_HeadLampSW_enum!=3)]
      (junction 2665) -> sNormal : [VPMM_PwrSta_enum>3||VINP_HeadLampSW_enum==3]
      AutoCutDetect -> (junction 2665) [order 1]
      AutoCut.Normal.AutoCut -> (junction 2665)
      AutoCutDetect -> AutoCut.Normal.AutoCut [order 2] : eLock
      AutoCutDetect -> AutoCut.Normal.AutoCut [order 3] : [after(4000,tick)]
      AutoCut.Normal.Unlock -> sNormal [order 2] : [VPMM_PwrSta_enum>3]
      (default) -> AutoCut.Normal.AutoCut
      AutoCut.Normal.Unlock -> AutoCut.Normal.AutoCut [order 1] : eLock
      AutoCut.Normal.Unlock -> AutoCut.Normal.AutoCut [order 3] : [after(3000,tick)]
      Normal -> AutoCut.Normal.Unlock [order 1] : eUnlock[VPMM_PwrSta_enum<=3]
    note: 4000
    note: 40 sec
    (default) -> Normal
    Normal -> FollowMeHome [order 1] : eFollow[VPMM_PwrSta_enum<=3]
    FollowMeHome -> sNormal [order 2] : eFollow
    FollowMeHome -> sNormal [order 3] : [VPMM_PwrSta_enum>3]
    FollowMeHome -> (junction 2717) [order 1] : [after(VBCM_DiagFMHT_s,tick)]
    (junction 2717) -> sNormal [order 1] : [VPMM_PwrSta_enum>3||...
        |  VINP_HeadLampSW_enum==3]
    (junction 2717) -> (junction 2719) [order 2]
    (junction 2719) -> AutoCut.Normal.AutoCut
  state LowBeam [parallel]
    settings: executionOrder=8
    state sLBeam
      en:VBCM_LBeam_flg=1;
    state sOFF
      en:VBCM_LBeam_flg=0;
    (default) -> LowBeam.sOFF
    (junction 2417) -> sLBeam [order 1] : [VBCM_HBeam_flg]
    LowBeam.sOFF -> (junction 2417) [order 1] : [!VBCM_AutoCut_flg]
    (junction 2417) -> (junction 2418) [order 2]
    (junction 2418) -> sLBeam [order 1] : [VINP_HeadLampSW_enum==2]
    (junction 2418) -> (junction 2419) [order 2]
    (junction 2419) -> sLBeam [order 1] : [VPMM_PwrSta_enum > VBCM_HLBeamENPwrSta_enum &&....
        | VINP_HeadLampSW_enum == 0 &&....
        | VINP_RLSLampSta_flg]
    (junction 2419) -> (junction 2420) [order 2]
    (junction 2420) -> sLBeam : [VBCM_FollowMe_flg]
    LowBeam.sOFF -> sLBeam [order 2] : [VBCM_showupEN_flg && VBCM_showup_flg]
    (junction 2421) -> LowBeam.sOFF [order 1] : [VBCM_AutoCut_flg]
    sLBeam -> (junction 2421) : [!VBCM_showupEN_flg || !VBCM_showup_flg]
    (junction 2421) -> (junction 2422) [order 2]
    (junction 2422) -> LowBeam.sOFF : [!VBCM_FollowMe_flg &&....
        | !VBCM_HBeam_flg &&....
        | VINP_HeadLampSW_enum != 2 &&....
        | (VINP_HeadLampSW_enum!=0 ||....
        | !VINP_RLSLampSta_flg ||....
        | VPMM_PwrSta_enum <= VBCM_HLBeamENPwrSta_enum)]
  state HighBeam [parallel]
    settings: executionOrder=7
    state sOFF
      en:VBCM_HBeam_flg=0;
    state sHBeam
      en:VBCM_HBeam_flg=1;
    (default) -> HighBeam.sOFF
    HighBeam.sOFF -> (junction 2455) : [!VBCM_AutoCut_flg]
    (junction 2455) -> sHBeam [order 1] : [VINP_CSWPassSWSta_flg]
    (junction 2455) -> (junction 2456) [order 2]
    (junction 2456) -> (junction 2457) : [VINP_CSWDimSw_flg]
    (junction 2457) -> sHBeam [order 1] : [VINP_HeadLampSW_enum==2]
    (junction 2457) -> (junction 2458) [order 2]
    (junction 2458) -> sHBeam : [VINP_HeadLampSW_enum == 0 &&....
        | VINP_RLSLampSta_flg == 1 &&....
        | VINP_ForceLowBeam_enum == 0 &&....
        | VPMM_PwrSta_enum > VBCM_HLBeamENPwrSta_enum &&....
        | VBCM_AutoHLB_flg]
    sHBeam -> HighBeam.sOFF [order 1] : [VBCM_AutoCut_flg]
    sHBeam -> (junction 2459) [order 2] : [!VINP_CSWPassSWSta_flg]
    (junction 2459) -> HighBeam.sOFF [order 1] : [!VINP_CSWDimSw_flg]
    (junction 2459) -> (junction 2605) [order 2]
    (junction 2605) -> (junction 2460) : [VINP_HeadLampSW_enum!=2]
    (junction 2460) -> HighBeam.sOFF [order 1] : [VINP_HeadLampSW_enum!=0]
    (junction 2460) -> (junction 2462) [order 2]
    (junction 2462) -> HighBeam.sOFF [order 1] : [VINP_RLSLampSta_flg==0 || VPMM_PwrSta_enum <= VBCM_HLBeamENPwrSta_enum]
    (junction 2462) -> (junction 2463) [order 2]
    (junction 2463) -> HighBeam.sOFF : [VINP_ForceLowBeam_enum==1||!VBCM_AutoHLB_flg]
  state AutoHLB [parallel]
    settings: executionOrder=13
    state AutoON
      on after(KBCM_ONDelayT_ms, tick):
      VBCM_AutoHLB_flg = TRUE;
    state AutoOFF
      en:
      VBCM_AutoHLB_flg = FALSE;
    (default) -> AutoOFF
    AutoOFF -> AutoON : [VINP_METERKPHCalcu_kph >= 30 && VINP_METERKPHCalcu_kph < 255]
    AutoON -> AutoOFF : [VINP_METERKPHCalcu_kph <= 25]
  state RBSD_CTRL [parallel]
    settings: executionOrder=10
    state OFF
      en:VBCM_RBSD_flg=0;
    state FlashOFF
      en:VBCM_RBSD_flg=0;
    state ON
      en:VBCM_RBSD_flg=1;
    (default) -> RBSD_CTRL.OFF
    RBSD_CTRL.FlashOFF -> RBSD_CTRL.OFF [order 1] : [VINP_SRRBSDWarnR_enum==0 && VINP_SRRODAWarnR_enum==0]
    RBSD_CTRL.ON -> RBSD_CTRL.FlashOFF [order 2] : [after(13,tick)&&(VINP_SRRBSDWarnR_enum==2||VINP_SRRODAWarnR_enum==2)]
    RBSD_CTRL.FlashOFF -> RBSD_CTRL.ON [order 2] : [after(12,tick)]
    RBSD_CTRL.ON -> RBSD_CTRL.OFF [order 1] : [VINP_SRRBSDWarnR_enum==0 && VINP_SRRODAWarnR_enum==0]
    RBSD_CTRL.OFF -> RBSD_CTRL.ON : [VINP_SRRBSDWarnR_enum>0 || VINP_SRRODAWarnR_enum>0]
  state LBSD_CTRL [parallel]
    settings: executionOrder=9
    state OFF
      en:VBCM_LBSD_flg=0;
    state FlashOFF
      en:VBCM_LBSD_flg=0;
    state ON
      en:VBCM_LBSD_flg=1;
    (default) -> LBSD_CTRL.OFF
    LBSD_CTRL.FlashOFF -> LBSD_CTRL.OFF [order 1] : [VINP_SRRBSDWarnL_enum==0 && VINP_SRRODAWarnL_enum==0]
    LBSD_CTRL.ON -> LBSD_CTRL.FlashOFF [order 2] : [after(13,tick)&&(VINP_SRRBSDWarnL_enum==2||VINP_SRRODAWarnL_enum==2)]
    LBSD_CTRL.FlashOFF -> LBSD_CTRL.ON [order 2] : [after(12,tick)]
    LBSD_CTRL.ON -> LBSD_CTRL.OFF [order 1] : [VINP_SRRBSDWarnL_enum==0 && VINP_SRRODAWarnL_enum==0]
    LBSD_CTRL.OFF -> LBSD_CTRL.ON : [VINP_SRRBSDWarnL_enum>0 || VINP_SRRODAWarnL_enum>0]
  data: VPMM_PwrSta_enum input uint8 [0..5]; VBCM_PwrStaBuf_enum input uint8; VINP_HeadLampSW_enum input uint8 [0..3]; VINP_RFogLampSW_flg input boolean; VINP_BrakeSWGPIO_flg input boolean; VINP_CSWDimSw_flg input boolean; VINP_CSWPassSWSta_flg input boolean; VTQD_ShiftGearPosn_enum input uint8 [0..15]; VBCM_PosLamp_flg output boolean; VBCM_LBeam_flg output boolean; VBCM_HBeam_flg output boolean; VBCM_RrFogLamp_flg output boolean; VBCM_BrakeLamp_flg output boolean; VBCM_ReverseLamp_flg output boolean; VBCM_OutMode_enum input uint8 [0..15]; VBCM_AutoCut_flg local boolean; VBCM_LDRL_flg output boolean; VBCM_RDRL_flg output boolean; VBCM_ATCtrl_enum input uint8 [0..2]; VINP_RLSLampSta_flg input boolean; VINP_ActBrkLampSta_flg input boolean; VINP_SRRODAWarnR_enum input; VINP_SRRODAWarnL_enum input; VINP_SRRBSDWarnR_enum input; VINP_SRRBSDWarnL_enum input; VINP_ForceLowBeam_enum input uint8; VTQD_ReBrakeLPReq_flg input; VBCM_LBSD_flg output boolean; VBCM_RBSD_flg output boolean; VBCM_DiagDRLOFF_flg input; VBCM_DiagFMHT_s input; ENUM_GEARPOSNTOCAN_P parameter; ENUM_POWERSTA_READY parameter; VBCM_showup_flg output boolean; VINP_METERKPHCalcu_kph input; KBCM_ONDelayT_ms input; VBCM_HLBeamENPwrSta_enum input; VBCM_showupEN_flg input; VBCM_FollowMe_flg output boolean; TRUE parameter; FALSE parameter; FDC_BCM_FollowMeENFun_Sta input; VBCM_AutoHLB_flg output boolean
  events: eLock local FUNCTION_CALL_EVENT; eUnlock local FUNCTION_CALL_EVENT; eFollow local FUNCTION_CALL_EVENT
